simulink model "erreurPo"  (R2017b)
settings: Solver=VariableStepAuto  StartTime=0.0  StopTime=2000  RelTol=1e-3
values from neighbouring files (symbols this model uses):
  Dep = Kp_ep.den{1}    [final2016.m]    (also in ordretwo.m)
  DPro = tfd3.den{1}    [final2016.m]    (also in ordretwo.m)
  Nep = Kp_ep.num{1}    [final2016.m]    (also in ordretwo.m)
  NPro = tfd3.num{1}    [final2016.m]    (also in ordretwo.m)
settings Model: Creator=lencs  LastModifiedBy=lencs

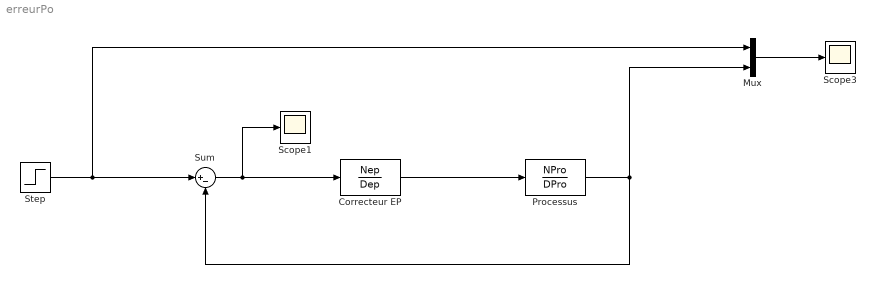
== system erreurPo ==
  Correcteur EP : DiscreteFilter  Numerator=Nep  Denominator=Dep  SampleTime=60
  Mux : Mux  Inputs=2
  Processus : DiscreteFilter  Numerator=NPro  Denominator=DPro  SampleTime=60
  Scope1 : Scope
  Scope3 : Scope
  Step : Step  SampleTime=0
  Sum : Sum  Inputs=|+-
  wires:
  Step/1 -> Mux/1, Sum/1
  Correcteur EP/1 -> Processus/1
  Sum/1 -> Scope1/1, Correcteur EP/1
  Processus/1 -> Sum/2, Mux/2
  Mux/1 -> Scope3/1
